simulink model "mx28_identification_p"  (R2014b)
settings: Solver=FixedStepDiscrete  StartTime=0.0  StopTime=5  RelTol=1e-3
undefined symbols (not defined in the file): darwinop_communication_setup
libraries: lib_darwinop x1
settings Model: SimulationMode=external  Creator=florent  LastModifiedBy=florent
settings OptimizationCC: OptimizeModelRefInitCode=on  LifeSpan=1
settings HardwareCC: ProdEndianess=LittleEndian  ProdHWDeviceType=Generic->32-bit Embedded Processor
settings RTWCC: SystemTargetFile=darwinoplib.tlc  GenCodeOnly=on  TemplateMakefile=darwinoplib.tmf  Description=DarwinOP code generator  ProcessScript=darwinoplib_make_rtw_hook  TargetLang=C++
settings CodeAppCC: IgnoreCustomStorageClasses=off
settings STFCustomTargetCC: CombineOutputUpdateFcns=on  ERTCustomFileBanners=on  SupportContinuousTime=off  SupportNonInlinedSFcns=off  MATLABClassNameForMDSCustomization=Simulink.SoftwareTarget.ERTCustomization  GRTInterface=off  SystemTargetFile=darwinoplib.tlc
settings ERTTargetCC: ParMdlRefBuildCompliant=off  CompOptLevelCompliant=off  ConcurrentExecutionCompliant=off  ERTFirstTimeCompliant=off  ModelStepFunctionPrototypeControlCompliant=off  CPPClassGenCompliant=off  ExtMode=on  ExtModeStaticAlloc=on  ExtModeStaticAllocSize=100000000  ExtModeMexArgs='192.168.123.1' 1 17725  InlinedParameterPlacement=NonHierarchical  ERTCustomFileTemplate=darwinoplib_main.tlc

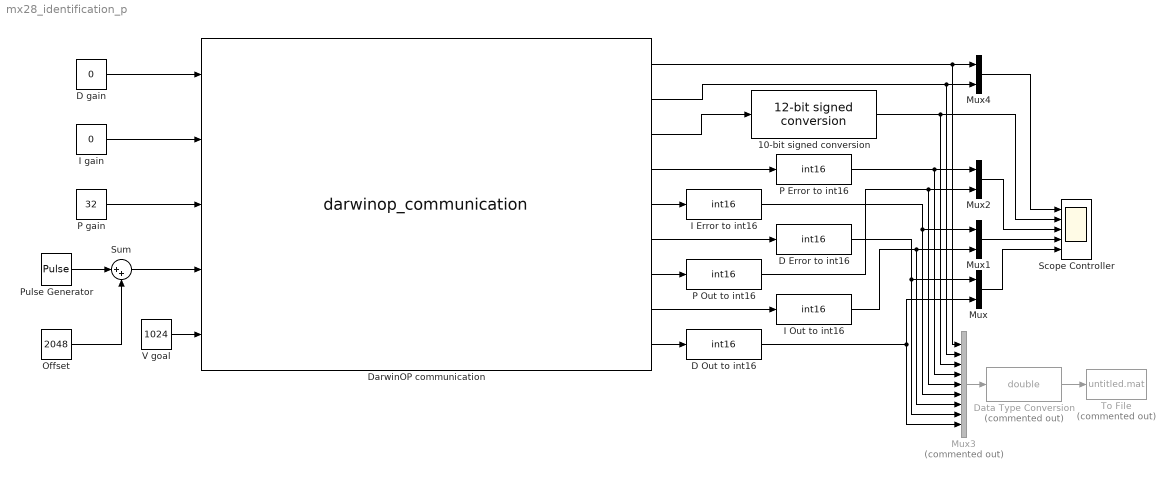
== system mx28_identification_p ==
  10-bit signed conversion : lib_darwinop/12-bit signed conversion
  D Error to int16 : DataTypeConversion  OutDataTypeStr=int16  ConvertRealWorld=Stored Integer (SI)
  D Out to int16 : DataTypeConversion  OutDataTypeStr=int16  ConvertRealWorld=Stored Integer (SI)
  D gain : Constant  Value=0
  DarwinOP communication : M-S-Function  StartFcn=darwinop_communication_setup('StartFcn');  StopFcn=darwinop_communication_setup('StopFcn');  FunctionName=darwinop_communication  Parameters=IP,Port,Protocol,SampleTime,Frame,ReadIndex,WriteIndex  mask{IP=192.168.123.1, Port=1234, Protocol=tcp, SampleTime=0.008, Frame=[ 2 1 30 2 2 1 36 2 2 1 54 14 3 1 26 3 0 0 0 3 1 30 4 0 0 0 0], ReadIndex=[ 1 2;3 2;5 2;7 2;9 2;11 2;13 2;15 2;17 2], WriteIndex=[ 17 1;18 1;19 1;24 2;26 2]}
      settings: DeleteFcn=darwinop_communication_setup('DeleteFcn');  ModelCloseFcn=darwinop_communication_setup('ModelCloseFcn');  NameChangeFcn=darwinop_communication_setup('NameChangeFcn');  OpenFcn=darwinop_communication_setup('OpenFcn');
      mask TypeOptions Protocol: tcp | udp
      mask Display:
      | image('darwin-blk.jpg')
      | 
      | port_label('output',1,'Épaule droite (tangage)(1)/Consigne de position')
      | port_label('output',2,'Épaule droite (tangage)(1)/Position courante')
      | port_label('output',3,'Épaule droite (tangage)(1)/PWM moteur')
      | port_label('output',4,'Épaule droite (tangage)(1)/Erreur P')
      | port_label('output',5,'Épaule droite (tangage)(1)/Erreur I')
      | port_label('output',6,'Épaule droite (tangage)(1)/Erreur D')
      | port_label('output',7,'Épaule droite (tangage)(1)/Commande P')
      | port_label('output',8,'Épaule droite (tangage)(1)/Commande I')
      | port_label('output',9,'Épaule droite (tangage)(1)/Commande D')
      | 
      | port_label('input',1,'Épaule droite (tangage)(1)/Gain D')
      | port_label('input',2,'Épaule droite (tangage)(1)/Gain I')
      | port_label('input',3,'Épaule droite (tangage)(1)/Gain P')
      | port_label('input',4,'Épaule droite (tangage)(1)/Consigne de position')
      | port_label('input',5,'Épaule droite (tangage)(1)/Consigne de vitesse')
  Data Type Conversion : DataTypeConversion  Commented=on  OutDataTypeStr=double
  I Error to int16 : DataTypeConversion  OutDataTypeStr=int16  ConvertRealWorld=Stored Integer (SI)
  I Out to int16 : DataTypeConversion  OutDataTypeStr=int16  ConvertRealWorld=Stored Integer (SI)
  I gain : Constant  Value=0
  Mux{,1..2,4} (4 alike) : Mux  Inputs=2
  Mux3 : Mux  Commented=on  Inputs=9
  Offset : Constant  Value=2048
  P Error to int16 : DataTypeConversion  OutDataTypeStr=int16  ConvertRealWorld=Stored Integer (SI)
  P Out to int16 : DataTypeConversion  OutDataTypeStr=int16  ConvertRealWorld=Stored Integer (SI)
  P gain : Constant  Value=32
  Pulse Generator : DiscretePulseGenerator  Amplitude=1024  Period=1000  PulseWidth=500  SampleTime=0.008
  Scope Controller : Scope  NumInputPorts=5
      settings: YMin=-5~-5~-5~-5~-5  YMax=5~5~5~5~5
  Sum : Sum  Inputs=|++
  To File : ToFile  Commented=on  MatrixName=Data
  V goal : Constant  Value=1024
  wires:
  P Error to int16/1 -> Mux3/4, Mux2/1
  I Error to int16/1 -> Mux3/6, Mux1/1
  D Error to int16/1 -> Mux3/8, Mux/1
  D Out to int16/1 -> Mux3/9, Mux/2
  I Out to int16/1 -> Mux3/7, Mux1/2
  P Out to int16/1 -> Mux3/5, Mux2/2
  Offset/1 -> Sum/2
  Pulse Generator/1 -> Sum/1
  Mux3/1 -> Data Type Conversion/1
  Data Type Conversion/1 -> To File/1
  V goal/1 -> DarwinOP communication/5
  P gain/1 -> DarwinOP communication/3
  I gain/1 -> DarwinOP communication/2
  D gain/1 -> DarwinOP communication/1
  10-bit signed conversion/1 -> Mux3/3, Scope Controller/2
  Mux/1 -> Scope Controller/5
  Mux1/1 -> Scope Controller/4
  Mux2/1 -> Scope Controller/3
  DarwinOP communication/9 -> D Out to int16/1
  DarwinOP communication/8 -> I Out to int16/1
  DarwinOP communication/7 -> P Out to int16/1
  DarwinOP communication/6 -> D Error to int16/1
  DarwinOP communication/5 -> I Error to int16/1
  DarwinOP communication/4 -> P Error to int16/1
  DarwinOP communication/3 -> 10-bit signed conversion/1
  DarwinOP communication/1 -> Mux3/1, Mux4/1
  DarwinOP communication/2 -> Mux3/2, Mux4/2
  Mux4/1 -> Scope Controller/1
  Sum/1 -> DarwinOP communication/4
